simulink model "assignment2"  (R2022b)
settings: Solver=VariableStepAuto  StartTime=0.0  StopTime=10.0  RelTol=1e-3
settings Model: Creator=user  LastModifiedBy=user

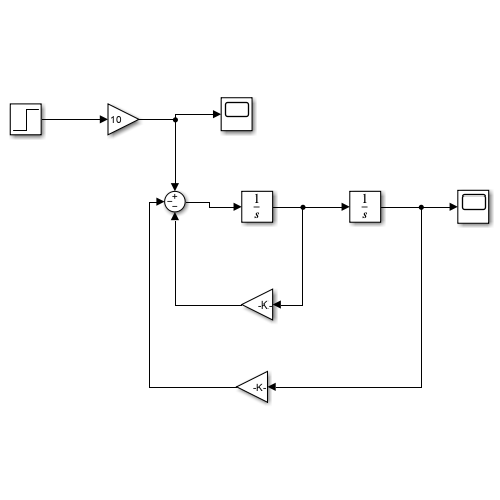
[thumbnail: Simulink's stored preview of the top-level diagram]
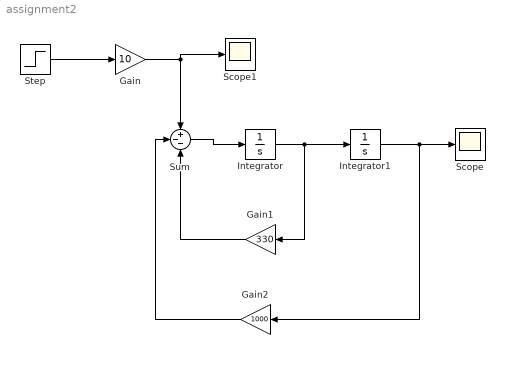
== system assignment2 ==
  Gain : Gain  Gain=10
  Gain1 : Gain  Gain=330
  Gain2 : Gain  Gain=1000
  Integrator : Integrator
  Integrator1 : Integrator
  Scope : Scope
  Scope1 : Scope
  Step : Step  SampleTime=0
  Sum : Sum  Inputs=+--
  wires:
  Step/1 -> Gain/1
  Gain/1 -> Sum/1, Scope1/1
  Sum/1 -> Integrator/1
  Gain1/1 -> Sum/3
  Gain2/1 -> Sum/2
  Integrator1/1 -> Gain2/1, Scope/1
  Integrator/1 -> Gain1/1, Integrator1/1
